simulink model "Demo_LQR_HSD_first"  (R2018b)
settings: Solver=ode1  StartTime=0.0  StopTime=20  FixedStep=0.001  MaxStep=0.001  RelTol=1e-3
InitFcn:
  | close all;
  | clc;
  | clear;
StopFcn:
  | position = system_output(:,1);
  | speed = system_output(:,2);
  | angle = system_output(:,3);
  | angular_velocity = system_output(:,4);
  | t = [1:length(position)];
  | 
  | figure;plot(t,position);
  | title('Position');
  | saveas(gcf,'Position.png');
  | figure;plot(t,speed);
  | title('Speed');
  | saveas(gcf,'speed.png');
  | figure;plot(t,angle);
  | title('Angle');
  | saveas(gcf,'angle.png');
  | figure;plot(t,angular_velocity);
  | title('Angle Velocity');
  | saveas(gcf,'angular_velocity.png');
  | 
  | u_law = control_output(:,1);
  | u_NN = control_output(:,2);
  | u_LQR = control_output(:,3);
  | t = [1:length(u_law)];
  | 
  | figure;plot(t,u_law);
  | title('u law');
  | saveas(gcf,'u_law.png');
  | figure;plot(t,u_NN);
  | title('u NN');
  | saveas(gcf,'u_NN.png');
  | figure;plot(t,u_LQR);
  | title('u LQR');
  | saveas(gcf,'u_LQR.png');
settings Model: Creator=Lenovo  LastModifiedBy=Richard
settings DataIOCC: LimitDataPoints=on  SaveFormat=Array
settings OptimizationCC: BlockReduction=off  BooleanDataType=off  LifeSpan=inf
settings DebuggingCC: SaveWithParameterizedLinksMsg=none  UnderspecifiedInitializationDetection=Classic  MergeDetectMultiDrivingBlocksExec=none  SignalResolutionControl=TryResolveAllWithWarning  SFUnexpectedBacktrackingDiag=warning  SFNoUnconditionalDefaultTransitionDiag=warning  SFExecutionAtInitializationDiag=none
settings HardwareCC: ProdBitPerPointer=32  ProdBitPerSizeT=32  ProdBitPerPtrDiffT=32  ProdLargestAtomicFloat=None  ProdIntDivRoundTo=Undefined  ProdEndianess=Unspecified  ProdWordSize=32  ProdHWDeviceType=32-bit Generic  TargetUnknown=on
settings ModelReferenceCC: PropagateSignalLabelsOutOfModel=off
settings SFSimCC: SimUseLocalCustomCode=off
settings RTWCC: RTWUseLocalCustomCode=off
settings CodeAppCC: StateflowObjectComments=on
settings GRTTargetCC: TargetLangStandard=C89/C90 (ANSI)  GeneratePreprocessorConditionals=Disable all
settings ConfigComp: CovMetricSettings=dw  CovHtmlReporting=on  CovSaveCumulativeToWorkspaceVar=on  CovSaveSingleToWorkspaceVar=on  CovExternalEMLEnable=off  CovSFcnEnable=off

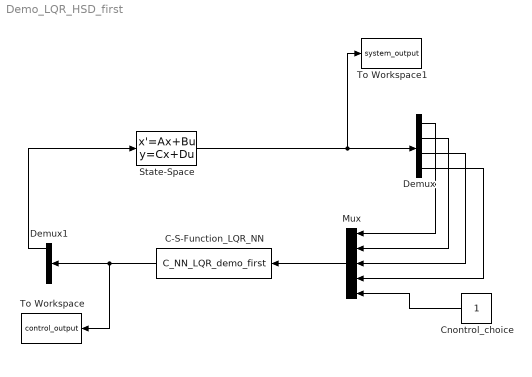
== system Demo_LQR_HSD_first ==
  C-S-Function_LQR_NN : S-Function  FunctionName=C_NN_LQR_demo_first  SFunctionDeploymentMode=off  EnableBusSupport=off
  Cnontrol_choice : Constant
  Demux : Demux
  Demux1 : Demux  Outputs=3
  Mux : Mux  Inputs=5
  State-Space : StateSpace  A=[0 1 0 0;0 -0.1164 1.2373 0;0 0 0 1;0 -0.7164 67.9221 0]  B=[0;1.4554;0;8.9546]  C=[1 0 0 0;0 1 0 0;0 0 1 0;0 0 0 1]  D=[0;0;0;0]  InitialCondition=[1;1;1;1]
  To Workspace : ToWorkspace  VariableName=control_output  SampleTime=-1
  To Workspace1 : ToWorkspace  VariableName=system_output  SampleTime=-1
  wires:
  Demux/1 -> Mux/1
  Demux/2 -> Mux/2
  Demux/4 -> Mux/4
  Mux/1 -> C-S-Function_LQR_NN/1
  Demux/3 -> Mux/3
  Demux1/1 -> State-Space/1
  Cnontrol_choice/1 -> Mux/5
  C-S-Function_LQR_NN/1 -> To Workspace/1, Demux1/1
  State-Space/1 -> To Workspace1/1, Demux/1
